simulink model "main"  (R2022b)
settings: Solver=VariableStepAuto  StartTime=0.0  StopTime=10.0  FixedStep=0.05  RelTol=1e-3
settings Model: Creator=pc  LastModifiedBy=pc

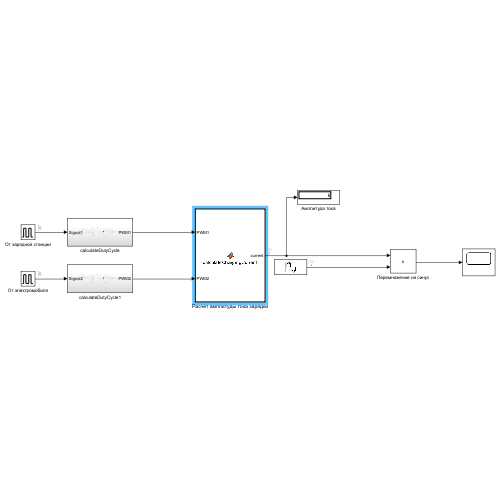
[thumbnail: Simulink's stored preview of the top-level diagram]
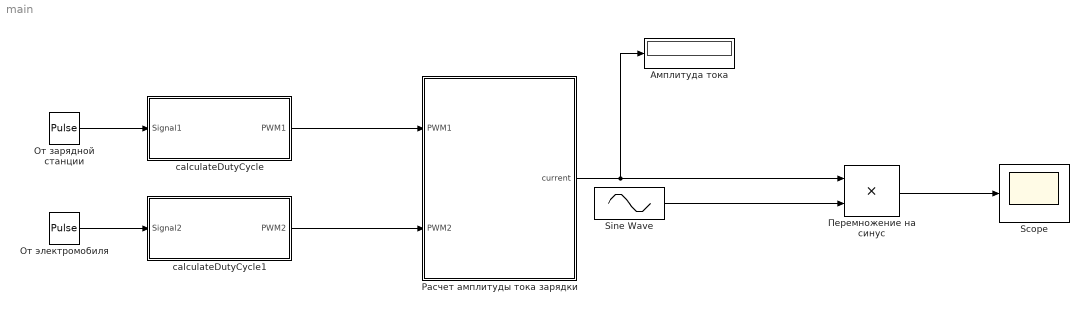
== system main ==
  Scope : Scope
  Sine Wave : Sin  Frequency=10  SampleTime=0.001
  calculateDutyCycle : Subsystem
  calculateDutyCycle1 : Subsystem
  Амплитуда тока : Display
  От зарядной станции : DiscretePulseGenerator  PulseType=Time based  Amplitude=5  Period=10  PulseWidth=90
  От электромобиля : DiscretePulseGenerator  PulseType=Time based  Amplitude=5  Period=10  PulseWidth=10
  Перемножение на синус : Product
  Расчет амплитуды тока зарядки : MATLAB Function  TreatAsAtomicUnit=on
  wires:
  Расчет амплитуды тока зарядки/1(current) -> Перемножение на синус/1, Амплитуда тока/1
  Sine Wave/1 -> Перемножение на синус/2
  Перемножение на синус/1 -> Scope/1
  От зарядной станции/1 -> calculateDutyCycle/1(Signal1)
  От электромобиля/1 -> calculateDutyCycle1/1(Signal2)
  calculateDutyCycle/1(PWM1) -> Расчет амплитуды тока зарядки/1(PWM1)
  calculateDutyCycle1/1(PWM2) -> Расчет амплитуды тока зарядки/2(PWM2)

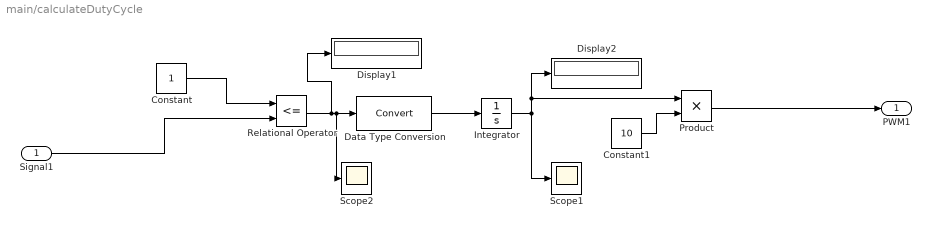
== system main/calculateDutyCycle ==
  Signal1 : Inport
  Constant : Constant
  Constant1 : Constant  Value=10
  Data Type Conversion : DataTypeConversion  SaturateOnIntegerOverflow=off  RndMeth=Floor
  Display1 : Display
  Display2 : Display
  Integrator : Integrator
  Product : Product
  Relational Operator : RelationalOperator  Operator=<=  OutDataTypeStr=boolean  RndMeth=Simplest  InputSameDT=off
  Scope1 : Scope
  Scope2 : Scope
  PWM1 : Outport
  wires:
  Integrator/1 -> Product/1, Display2/1, Scope1/1
  Constant/1 -> Relational Operator/1
  Relational Operator/1 -> Display1/1, Scope2/1, Data Type Conversion/1
  Data Type Conversion/1 -> Integrator/1
  Signal1/1 -> Relational Operator/2
  Constant1/1 -> Product/2
  Product/1 -> PWM1/1

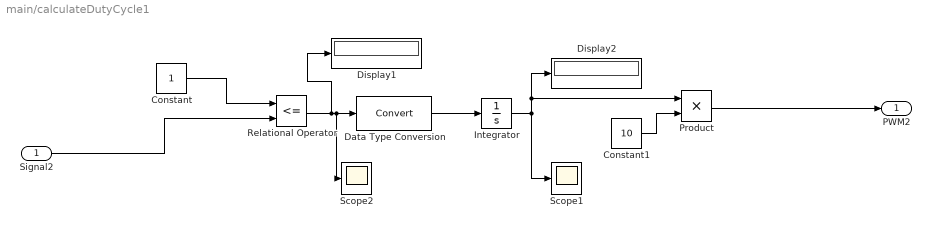
== system main/calculateDutyCycle1 ==
  Signal2 : Inport
  Constant : Constant
  Constant1 : Constant  Value=10
  Data Type Conversion : DataTypeConversion  SaturateOnIntegerOverflow=off  RndMeth=Floor
  Display1 : Display
  Display2 : Display
  Integrator : Integrator
  Product : Product
  Relational Operator : RelationalOperator  Operator=<=  OutDataTypeStr=boolean  RndMeth=Simplest  InputSameDT=off
  Scope1 : Scope
  Scope2 : Scope
  PWM2 : Outport
  wires:
  Integrator/1 -> Product/1, Display2/1, Scope1/1
  Constant/1 -> Relational Operator/1
  Relational Operator/1 -> Display1/1, Scope2/1, Data Type Conversion/1
  Data Type Conversion/1 -> Integrator/1
  Signal2/1 -> Relational Operator/2
  Constant1/1 -> Product/2
  Product/1 -> PWM2/1

== matlab function main/Расчет амплитуды тока зарядки ==
  data: PWM1 input; current output; PWM2 input
function current = calculateChargingCurrent(PWM1, PWM2)
    % PWM1 - входное значение ШИМ от зарядной станции (от 0 до 100)
    % PWM2 - входное значение ШИМ от электромобиля (от 0 до 100)
    % current - выходное значение тока зарядки

    % Инициализация переменных
    current1 = 0;
    current2 = 0;

    % Расчет тока, который может выдавать зарядная станция
    if PWM1 < 5
        % Зарядка запрещена
        current1 = 0;
    elseif PWM1 >= 5 && PWM1 < 10
        % Ожидание цифровой коммуникации
        current1 = 0;
    elseif PWM1 >= 10 && PWM1 <= 85
        % Ток зарядки = (% цикла * 100) * 0.6 А
        current1 = PWM1 * 0.6;
    elseif PWM1 > 85 && PWM1 <= 90
        % Ток зарядки = (% цикла * 100 - 64) * 2.5 А, но не более 63 А
        current1 = (PWM1 * 100 - 64) * 2.5;
        current1 = min(current1, 63); % Ограничение до 63 А
    elseif PWM1 > 90 && PWM1 <= 97
        % Зарезервировано (зарядка запрещена)
        current1 = 0;
    else
        % Зарядка запрещена
        current1 = 0;
    end

    % Расчет тока, который может принимать электромобиль
    if PWM2 < 3
        % Зарядка запрещена
        current2 = 0;
    elseif PWM2 >= 3 && PWM2 < 7
        % Ожидание цифровой коммуникации
        current2 = 0;
    elseif PWM2 >= 7 && PWM2 <= 8
        % Зарядка запрещена
        current2 = 0;
    elseif PWM2 >= 8 && PWM2 <= 10
        % Ток зарядки = 6 А
        current2 = 6;
    elseif PWM2 >= 10 && PWM2 <= 85
        % Ток зарядки = (% цикла * 100) * 0.6 А
        current2 = PWM2 * 0.6;
    elseif PWM2 > 85 && PWM2 <= 90
        % Ток зарядки = (% цикла * 100 - 64) * 2.5 А
        current2 = (PWM2 * 100 - 64) * 2.5;
    elseif PWM2 > 90 && PWM2 <= 97
        % Зарезервировано (зарядка запрещена)
        current2 = 0;
    else
        % Зарядка запрещена
        current2 = 0;
    end

    % Определение итогового тока зарядки
    if current1 > 0 && current2 > 0
        % Ток зарядки ограничивается минимальным значением
        current = min(current1, current2);
    else
        % Если один из токов равен нулю, зарядка запрещена
        current = 0;
    end
end
